simulink model "simulation_servo_agent"  (R2017b)
settings: Solver=FixedStepDiscrete  StartTime=0.0  StopTime=inf  FixedStep=Ts  MaxStep=1e-2  RelTol=1e-3  AbsTol=1e-3
PreLoadFcn:
  | pe_dc_motor_control_data;
values from neighbouring files (symbols this model uses):
  K = 0.00648887065107    [best_params.mat]    (also in parameter_twiddle_fast_kr.m = params(1))
  R = 5.66592438851    [best_params.mat]    (also in parameter_twiddle_fast_kr.m = params(2))
  Ts = 0.001    [best_params.mat]
undefined symbols (not defined in the file or in its folder): RawAcceleration, RawCurrent, RawPwm, RawRequestedVelocity, RawSupplyVoltage, RawTemperature, RawTimestamp, RawTorque, RawVelocity
libraries: fl_lib x21, nesl_utility x10, robotlib x8, dspstat3 x2, simulink x1, powerlib_meascontrol x1, commchan3 x1, sdl_lib x1
Description:
  | DC Motor Control
  | 
  | This example shows a cascade speed-control structure for a DC motor.
  | A PWM controlled four-quadrant Chopper is used to feed the DC motor.
  | The Control subsystem includes the outer speed-control loop, the inner
  | current-control loop, and the PWM generation. The total simulation
  | time (t) is 4 seconds. At t = 1.5 seconds, the load torque increases.
  | At t = 2.5 seconds, the reference speed is changed from 1000 rpm to
  | 2000 rpm.
  | 
  | Copyright 2016-2017 The MathWorks, Inc.
settings Model: Creator=The MathWorks, Inc.  LastModifiedBy=s158031
settings OptimizationCC: EnhancedBackFolding=on  PassReuseOutputArgsThreshold=0  MaxStackSize=64  OptimizeBlockOrder=speed  DifferentSizesBufferReuse=on
settings DebuggingCC: UnderspecifiedInitializationDetection=Classic  MergeDetectMultiDrivingBlocksExec=none  ParameterTunabilityLossMsg=error  SFUnexpectedBacktrackingDiag=warning  SFNoUnconditionalDefaultTransitionDiag=warning  SFExecutionAtInitializationDiag=none
settings HardwareCC: ProdBitPerPointer=32  ProdBitPerSizeT=32  ProdBitPerPtrDiffT=32  ProdLargestAtomicFloat=None  ProdIntDivRoundTo=Undefined  ProdEndianess=Unspecified  ProdWordSize=32  ProdHWDeviceType=Generic->Unspecified (assume 32-bit Generic)
settings SFSimCC: MATLABDynamicMemAlloc=off
settings RTWCC: SystemTargetFile=ert.tlc  HardwareBoard=Robot Operating System (ROS)  TemplateMakefile=ert_default_tmf  GenerateReport=on  Toolchain=Catkin  LaunchReport=on  TargetLang=C++
settings CodeAppCC: ForceParamTrailComments=on  OperatorAnnotations=on
settings ERTTargetCC: ERTCustomFileBanners=off  SupportContinuousTime=on  SupportNonInlinedSFcns=on  RemoveResetFunc=off  ModelStepFunctionPrototypeControlCompliant=off
settings ConfigComp: CovMetricSettings=dw  CovHtmlReporting=on  CovSaveCumulativeToWorkspaceVar=on  CovSaveSingleToWorkspaceVar=on  CovExternalEMLEnable=off
settings SimscapeCC: SimscapeLogName=simlog_pe_dc_motor_control  SimscapeLogLimitData=off

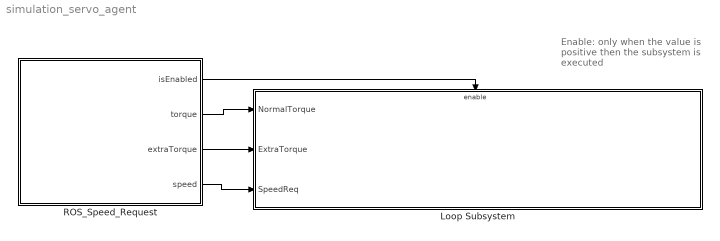
== system simulation_servo_agent ==
  note: Enable: only when the value is positive then the subsystem is executed
  Loop Subsystem : Subsystem
  ROS_Speed_Request : Subsystem
  wires:
  ROS_Speed_Request/2(torque) -> Loop Subsystem/1("NormalTorque ")
  ROS_Speed_Request/1(isEnabled) -> Loop Subsystem/Enable
  ROS_Speed_Request/3(extraTorque) -> Loop Subsystem/2(ExtraTorque)
  ROS_Speed_Request/4(speed) -> Loop Subsystem/3(SpeedReq)

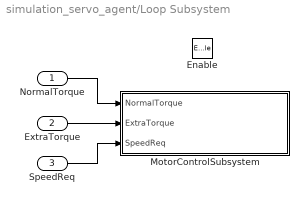
== system simulation_servo_agent/Loop Subsystem ==
  "NormalTorque " : Inport
  ExtraTorque : Inport  Port=2
  SpeedReq : Inport  Port=3
  Enable : EnablePort
  MotorControlSubsystem : Subsystem  TreatAsAtomicUnit=on
  wires:
  "NormalTorque "/1 -> MotorControlSubsystem/1(NormalTorque)
  SpeedReq/1 -> MotorControlSubsystem/3(SpeedReq)
  ExtraTorque/1 -> MotorControlSubsystem/2(ExtraTorque)

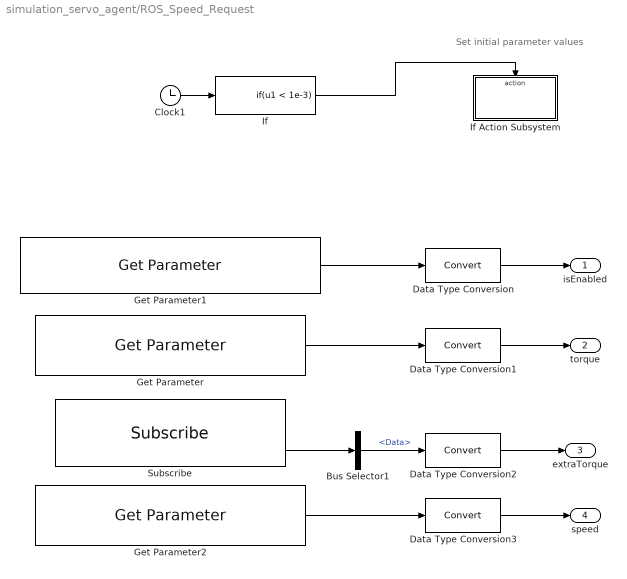
== system simulation_servo_agent/ROS_Speed_Request ==
  note: Set initial parameter values
  Bus Selector1 : BusSelector  OutputSignals=Data
  Clock1 : Clock
  Data Type Conversion{,1..3} (4 alike) : DataTypeConversion
  Get Parameter : robotlib/Get Parameter  SourceLibraryInfo=This block requires Robotics System Toolbox  ParameterSource=Select from ROS network  ParameterName=/simulation_servo_agent/add_torque/torque  ParameterType=double  ParameterMaxArrayLength=16  ParameterInitialValue=0.0  SampleTime=-1  ShowErrorCodeOutput=off  ModelName=simulation_servo_agent  BlockId=ParamGet_simulation_servo_agent_3318
      settings: SourceProductName=Robotics System Toolbox  SourceProductBaseCode=RO
  Get Parameter1 : robotlib/Get Parameter  SourceLibraryInfo=This block requires Robotics System Toolbox  ParameterSource=Select from ROS network  ParameterName=/simulation_servo_agent/update_velocity/isEnabled  ParameterType=boolean  ParameterMaxArrayLength=16  ParameterInitialValue=0.0  SampleTime=-1  ShowErrorCodeOutput=off  ModelName=simulation_servo_agent  BlockId=ParamGet_simulation_servo_agent_3398
      settings: SourceProductName=Robotics System Toolbox  SourceProductBaseCode=RO
  Get Parameter2 : robotlib/Get Parameter  SourceLibraryInfo=This block requires Robotics System Toolbox  ParameterSource=Select from ROS network  ParameterName=/simulation_servo_agent/update_velocity/speed  ParameterType=double  ParameterMaxArrayLength=16  ParameterInitialValue=0.0  SampleTime=-1  ShowErrorCodeOutput=off  ModelName=simulation_servo_agent  BlockId=ParamGet_simulation_servo_agent_3752
      settings: SourceProductName=Robotics System Toolbox  SourceProductBaseCode=RO
  If : If  IfExpression=u1 < 1e-3  ShowElse=off
  If Action Subsystem : Subsystem  TreatAsAtomicUnit=on
  Subscribe : robotlib/Subscribe  SourceLibraryInfo=This block requires Robotics System Toolbox  topicSource=Select from ROS network  topic=/conveyor_belt_agent/extra_torque  messageType=std_msgs/Float32  sampleTime=-1  messageQueueLength=1
      settings: SourceProductBaseCode=RO
  isEnabled : Outport
  torque : Outport  Port=2
  extraTorque : Outport  Port=3
  speed : Outport  Port=4
  wires:
  Get Parameter/1 -> Data Type Conversion1/1
  Get Parameter1/1 -> Data Type Conversion/1
  Data Type Conversion/1 -> isEnabled/1
  Clock1/1 -> If/1
  If/1 -> If Action Subsystem/Action
  Data Type Conversion1/1 -> torque/1
  Data Type Conversion3/1 -> speed/1
  Get Parameter2/1 -> Data Type Conversion3/1
  Subscribe/2 -> Bus Selector1/1
  Bus Selector1/1 -> Data Type Conversion2/1  "<Data>"
  Data Type Conversion2/1 -> extraTorque/1

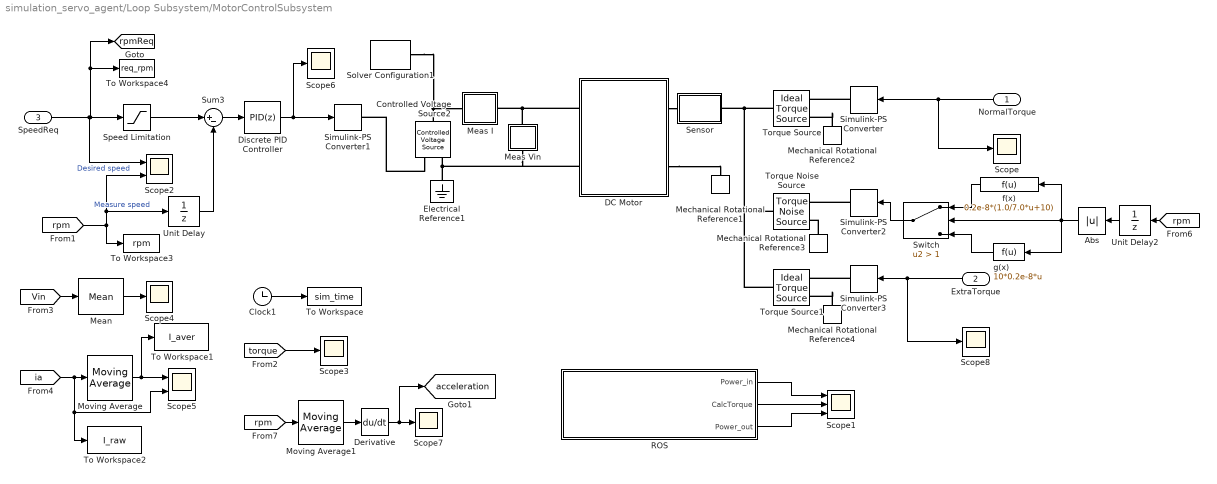
== system simulation_servo_agent/Loop Subsystem/MotorControlSubsystem ==
  NormalTorque : Inport
  ExtraTorque : Inport  Port=2
  SpeedReq : Inport  Port=3
  Abs : Abs
  Clock1 : Clock
  Controlled Voltage Source2 : fl_lib/Electrical/Electrical Sources/Controlled Voltage Source
  DC Motor : Subsystem
  Derivative : Derivative
  Discrete PID Controller : simulink/Continuous/PID Controller  Controller=PID  TimeDomain=Discrete-time  SampleTime=-1  IntegratorMethod=Forward Euler  FilterMethod=Forward Euler  Form=Parallel  UseFilter=on  ControllerParametersSource=internal  P=0.12  I=1.5  D=0.007  N=55  InitialConditionSource=internal  InitialConditionForIntegrator=0  InitialConditionForFilter=0  ExternalReset=none  LimitOutput=on  UpperSaturationLimit=11.1  LowerSaturationLimit=-11.1  LinearizeAsGain=off  AntiWindupMode=none  Kb=1  TrackingMode=off  Kt=1  PParamMin=[]  PParamMax=[]  IParamMin=[]  IParamMax=[]  DParamMin=[]  DParamMax=[]  NParamMin=[]  NParamMax=[]  KbParamMin=[]  KbParamMax=[]  KtParamMin=[]  KtParamMax=[]  POutMin=[]  POutMax=[]  IOutMin=[]  IOutMax=[]  DOutMin=[]  DOutMax=[]  NOutMin=[]  NOutMax=[]  KbOutMin=[]  KbOutMax=[]  KtOutMin=[]  KtOutMax=[]  IntegratorOutMin=[]  IntegratorOutMax=[]  FilterOutMin=[]  FilterOutMax=[]  SumOutMin=[]  SumOutMax=[]  SumI1OutMin=[]  SumI1OutMax=[]  SumI2OutMin=[]  SumI2OutMax=[]  SumI3OutMin=[]  SumI3OutMax=[]  SumDOutMin=[]  SumDOutMax=[]  SaturationOutMin=[]  SaturationOutMax=[]  IntegratorContinuousStateAttributes=''  IntegratorStateMustResolveToSignalObject=off  IntegratorRTWStateStorageClass=Auto  FilterContinuousStateAttributes=''  FilterStateMustResolveToSignalObject=off  FilterRTWStateStorageClass=Auto  DifferentiatorICPrevScaledInput=0  DifferentiatorOutMin=[]  DifferentiatorOutMax=[]  InitialConditionSetting=State (most efficient)  FilterDiffOutCoefMin=[]  FilterDiffOutCoefMax=[]  SumDenOutMin=[]  SumDenOutMax=[]  SumNumOutMin=[]  SumNumOutMax=[]  ReciprocalOutMin=[]  ReciprocalOutMax=[]  DivideOutMin=[]  DivideOutMax=[]  TunerSelectOption=Transfer Function Based (PID Tuner App)
  Electrical Reference1 : fl_lib/Electrical/Electrical Elements/Electrical Reference
      settings: SourceProductName=Foundation Library
  Mean : powerlib_meascontrol/Measurements/Mean  Freq=10  Vinit=0  Ts=Ts
  Meas I : Subsystem
  Meas Vin : Subsystem
  Mechanical Rotational Reference{1..4} (4 alike) : fl_lib/Mechanical/Rotational Elements/Mechanical Rotational Reference
      settings: SourceProductName=Foundation Library
  Moving Average : dspstat3/Moving Average  Method=Sliding window  SpecifyWindowLength=on  WindowLength=1000  ForgettingFactor=0.9  SimulateUsing=Code generation
  Moving Average1 : dspstat3/Moving Average  Method=Sliding window  SpecifyWindowLength=on  WindowLength=300  ForgettingFactor=0.9  SimulateUsing=Code generation
  ROS : Subsystem
  Scope{,3..4,6..8} (6 alike) : Scope
  Scope1 : Scope  NumInputPorts=3
  Scope2 : Scope  NumInputPorts=2
  Scope5 : Scope  NumInputPorts=2
  Sensor : Subsystem
  Simulink-PS Converter{,1..3} (4 alike) : nesl_utility/Simulink-PS Converter  PhysicalDomain=network_engine_domain  SubClassName=ps_input  LeftPortType=input  RightPortType=output  PseudoPeriodic=off  Frequencies=[]  NoiseDistribution=none  NoiseParameters=[]  Unit=1  AffineConversion=off  FilteringAndDerivatives=provide  SimscapeFilterOrder=1  InputFilterTimeConstant=0.001  UdotUserProvided=0
  Solver Configuration1 : nesl_utility/Solver Configuration  PhysicalDomain=network_engine_domain  SubClassName=solver  LeftPortType=input  RightPortType=generic  Accelerate=off  Tones=[]  Harmonics=[]  SimulateNoise=off  Profile=off  UseLocalSampling=off  EnableSwitchedLinearOptims=on  FrequencyDomain=off  UseCCode=off  RelTol=0.001  AbsTol=1e-06  MinStep=1e-09  ToWorkspace=off  RevertToSquareIcSolve=off  NumHomotopyIterations=100  PhasorMode=off  PhasorModeNumHarmonics=1  DoDC=off  ResidualTolerance=1e-09  UseLocalSolver=on  LocalSolverChoice=NE_BACKWARD_EULER_ADVANCER  LocalSolverSampleTime=Ts  DoFixedCost=on  MaxNonlinIter=3  MaxModeIter=2  LinearAlgebra=Sparse  DelaysMemoryBudget=1024  AutomaticFiltering=on  FilteringTimeConstant=0.001
  Speed Limitation : Saturate  UpperLimit=57  LowerLimit=-57
  Sum3 : Sum  Inputs=|+-
  Switch : Switch  Criteria=u2 > Threshold  Threshold=1
  To Workspace : ToWorkspace  VariableName=sim_time  SampleTime=-1
      settings: Save2DSignal=2-D array (concatenate along first dimension)
  To Workspace1 : ToWorkspace  VariableName=I_aver  SampleTime=-1
      settings: Save2DSignal=2-D array (concatenate along first dimension)
  To Workspace2 : ToWorkspace  VariableName=I_raw  SampleTime=-1
  To Workspace3 : ToWorkspace  VariableName=rpm  SampleTime=-1
      settings: Save2DSignal=2-D array (concatenate along first dimension)
  To Workspace4 : ToWorkspace  VariableName=req_rpm  SampleTime=-1
      settings: Save2DSignal=2-D array (concatenate along first dimension)
  Torque Source : fl_lib/Mechanical/Mechanical Sources/Ideal Torque Source
      settings: SourceProductName=Foundation Library
  Torque Source1 : fl_lib/Mechanical/Mechanical Sources/Ideal Torque Source
      settings: SourceProductName=Foundation Library
  Torque Noise Source : sdl_lib/Sources/Torque Noise Source  sample_time=1e-3 s  repeatability=3  user_seed=0  auto_seed=0
      settings: SourceProductName=Simscape Driveline  SourceProductBaseCode=LD
  Unit Delay : UnitDelay  SampleTime=Ts
  Unit Delay2 : UnitDelay  SampleTime=Ts
  f(x) : Fcn  Expr=0.2e-8*(1.0/7.0*u+10)
  g(x) : Fcn  Expr=10*0.2e-8*u
  tag scope: acceleration=global, rpmReq=global
  wires:
  NormalTorque/1 -> Simulink-PS Converter/1, Scope/1
  ROS/2(CalcTorque) -> Scope1/2
  ROS/1("Power_in ") -> Scope1/1
  ROS/3(Power_out) -> Scope1/3
  [Vin] -> Mean/1
  [ia] -> To Workspace2/1, Scope5/2, Moving Average/1
  Moving Average/1 -> To Workspace1/1, Scope5/1
  Mean/1 -> Scope4/1
  [rpm] -> To Workspace3/1, Unit Delay/1, Scope2/2  "Measure speed"
  Unit Delay/1 -> Sum3/2
  Clock1/1 -> To Workspace/1
  [torque] -> Scope3/1
  Speed Limitation/1 -> Sum3/1
  Sum3/1 -> Discrete PID Controller/1
  SpeedReq/1 -> [rpmReq], To Workspace4/1, Speed Limitation/1, Scope2/1  "Desired speed"
  Discrete PID Controller/1 -> Scope6/1, Simulink-PS Converter1/1
  [rpm] -> Moving Average1/1
  Derivative/1 -> [acceleration], Scope7/1
  Moving Average1/1 -> Derivative/1
  ExtraTorque/1 -> Scope8/1, Simulink-PS Converter3/1
  Switch/1 -> Simulink-PS Converter2/1
  f(x)/1 -> Switch/1
  [rpm] -> Unit Delay2/1
  Unit Delay2/1 -> Abs/1
  Abs/1 -> g(x)/1, f(x)/1, Switch/2
  g(x)/1 -> Switch/3
  connections:
  Meas Vin/LConn1 -- DC Motor/LConn1 -- Meas I/RConn1
  DC Motor/RConn1 -- Sensor/LConn1
  Simulink-PS Converter/RConn1 -- Torque Source/RConn1
  DC Motor/RConn2 -- Mechanical Rotational Reference1/LConn1
  Mechanical Rotational Reference2/LConn1 -- Torque Source/RConn2
  Electrical Reference1/LConn1 -- Controlled Voltage Source2/RConn2 -- DC Motor/LConn2 -- Meas Vin/RConn1
  Controlled Voltage Source2/LConn1 -- Solver Configuration1/RConn1 -- Meas I/LConn1
  Controlled Voltage Source2/RConn1 -- Simulink-PS Converter1/RConn1
  Torque Source/LConn1 -- Sensor/RConn1 -- Torque Source1/LConn1 -- Torque Noise Source/RConn1
  Simulink-PS Converter2/RConn1 -- Torque Noise Source/LConn1
  Mechanical Rotational Reference3/LConn1 -- Torque Noise Source/LConn2
  Simulink-PS Converter3/RConn1 -- Torque Source1/RConn1
  Mechanical Rotational Reference4/LConn1 -- Torque Source1/RConn2

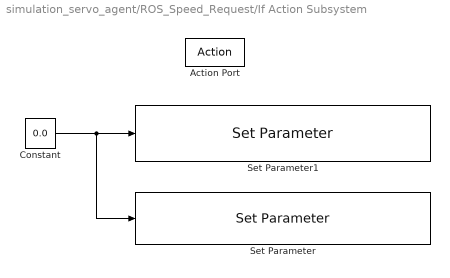
== system simulation_servo_agent/ROS_Speed_Request/If Action Subsystem ==
  Action Port : ActionPort  ActionType=then
  Constant : Constant  Value=0.0
  Set Parameter : robotlib/Set Parameter  SourceLibraryInfo=This block requires Robotics System Toolbox  ParameterSource=Select from ROS network  ParameterName=/simulation_servo_agent/update_velocity/isEnabled  ParameterType=double  ModelName=simulation_servo_agent  BlockId=ParamSet_simulation_servo_agent_3446
      settings: SourceProductName=Robotics System Toolbox  SourceProductBaseCode=RO
  Set Parameter1 : robotlib/Set Parameter  SourceLibraryInfo=This block requires Robotics System Toolbox  ParameterSource=Select from ROS network  ParameterName=/simulation_servo_agent/update_velocity/speed  ParameterType=double  ModelName=simulation_servo_agent  BlockId=ParamSet_simulation_servo_agent_3447
      settings: SourceProductName=Robotics System Toolbox  SourceProductBaseCode=RO
  wires:
  Constant/1 -> Set Parameter/1, Set Parameter1/1

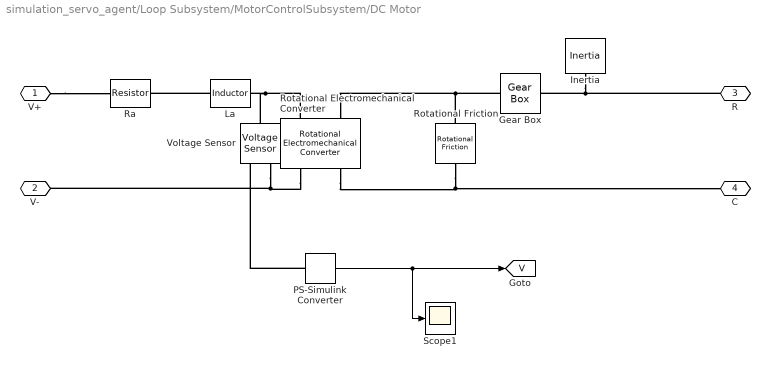
== system simulation_servo_agent/Loop Subsystem/MotorControlSubsystem/DC Motor ==
  Gear Box : fl_lib/Mechanical/Mechanisms/Gear Box  ratio=258.5  t_in_specify=off  t_in_priority=None  t_in=0 N*m  t_in_nominal_specify=off  t_in_nominal_unit=N*m  t_in_nominal_value=1  t_out_specify=off  t_out_priority=None  t_out=0 N*m  t_out_nominal_specify=off  t_out_nominal_unit=N*m  t_out_nominal_value=1
  Inertia : fl_lib/Mechanical/Rotational Elements/Inertia  inertia=J kg*m^2  w_specify=off  w_priority=High  w=0 rad/s  w_nominal_specify=off  w_nominal_unit=rad/s  w_nominal_value=1  t_specify=off  t_priority=None  t=0 N*m  t_nominal_specify=off  t_nominal_unit=N*m  t_nominal_value=1
      settings: SourceProductName=Foundation Library
  La : fl_lib/Electrical/Electrical Elements/Inductor  l=L H  r=0 Ohm  g=1e-9 1/Ohm  i_specify=off  i_priority=None  i=0 A  i_nominal_specify=off  i_nominal_unit=A  i_nominal_value=1  v_specify=off  v_priority=None  v=0 V  v_nominal_specify=off  v_nominal_unit=V  v_nominal_value=1  i_L_specify=on  i_L_priority=High  i_L=0 A  i_L_nominal_specify=off  i_L_nominal_unit=A  i_L_nominal_value=1
      settings: SourceProductName=Foundation Library
  PS-Simulink Converter : nesl_utility/PS-Simulink Converter  PhysicalDomain=network_engine_domain  SubClassName=ps_output  LeftPortType=input  RightPortType=output  PseudoPeriodic=off  Frequencies=[]  Unit=1  AffineConversion=off
  Ra : fl_lib/Electrical/Electrical Elements/Resistor  R=R Ohm  i_specify=off  i_priority=None  i=0 A  i_nominal_specify=off  i_nominal_unit=A  i_nominal_value=1  v_specify=off  v_priority=None  v=0 V  v_nominal_specify=off  v_nominal_unit=V  v_nominal_value=1
      settings: SourceProductName=Foundation Library
  Rotational Electromechanical Converter : fl_lib/Electrical/Electrical Elements/Rotational Electromechanical Converter  K=K V/(rad/s)  i_specify=off  i_priority=None  i=0 A  i_nominal_specify=off  i_nominal_unit=A  i_nominal_value=1  v_specify=off  v_priority=None  v=0 V  v_nominal_specify=off  v_nominal_unit=V  v_nominal_value=1  t_specify=off  t_priority=None  t=0 N*m  t_nominal_specify=off  t_nominal_unit=N*m  t_nominal_value=1  w_specify=off  w_priority=None  w=0 rad/s  w_nominal_specify=off  w_nominal_unit=rad/s  w_nominal_value=1
      settings: SourceProductName=Foundation Library
  Rotational Friction : fl_lib/Mechanical/Rotational Elements/Rotational Friction  brkwy_trq=C N*m  brkwy_vel=1e-5 rad/s  Col_trq=C N*m  visc_coef=F N*m/(rad/s)  w_specify=off  w_priority=None  w=0 rad/s  w_nominal_specify=off  w_nominal_unit=rad/s  w_nominal_value=1  t_specify=off  t_priority=None  t=0 N*m  t_nominal_specify=off  t_nominal_unit=N*m  t_nominal_value=1
      settings: SourceProductName=Simscape
  Scope1 : Scope
  Voltage Sensor : fl_lib/Electrical/Electrical Sensors/Voltage Sensor
  V+ : PMIOPort  Port=1  Side=Left
  V- : PMIOPort  Port=2  Side=Left
  R : PMIOPort  Port=3  Side=Right
  C : PMIOPort  Port=4  Side=Right
  tag scope: V=global
  wires:
  PS-Simulink Converter/1 -> Scope1/1, [V]
  connections:
  Rotational Electromechanical Converter/RConn1 -- Voltage Sensor/RConn2 -- V-/RConn1
  V+/RConn1 -- Ra/LConn1
  Rotational Electromechanical Converter/RConn2 -- Rotational Friction/RConn1 -- C/RConn1
  Gear Box/LConn1 -- Rotational Electromechanical Converter/LConn2 -- Rotational Friction/LConn1
  R/RConn1 -- Inertia/LConn1 -- Gear Box/RConn1
  Rotational Electromechanical Converter/LConn1 -- Voltage Sensor/LConn1 -- La/RConn1
  La/LConn1 -- Ra/RConn1
  PS-Simulink Converter/LConn1 -- Voltage Sensor/RConn1

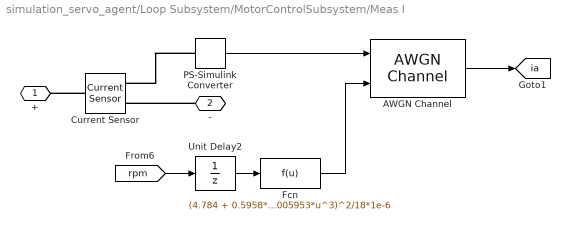
== system simulation_servo_agent/Loop Subsystem/MotorControlSubsystem/Meas I ==
  AWGN Channel : commchan3/AWGN Channel  InputProcessing=Columns as channels (frame based)  seed=67  noiseMode=Variance from port  EbNodB=10  EsNodB=10  SNRdB=10  bitsPerSym=1  Ps=1  Tsym=1  variance=1
  Current Sensor : fl_lib/Electrical/Electrical Sensors/Current Sensor
      settings: SourceProductName=Foundation Library
  Fcn : Fcn  Expr=(4.784 + 0.5958*u -0.02393*u^2+0.0005953*u^3)^2/18*1e-6
  PS-Simulink Converter : nesl_utility/PS-Simulink Converter  PhysicalDomain=network_engine_domain  SubClassName=ps_output  LeftPortType=input  RightPortType=output  PseudoPeriodic=off  Frequencies=[]  Unit=1  AffineConversion=off
  Unit Delay2 : UnitDelay  SampleTime=Ts
  + : PMIOPort  Port=1  Side=Left
  - : PMIOPort  Port=2  Side=Right
  tag scope: ia=global
  wires:
  AWGN Channel/1 -> [ia]
  [rpm] -> Unit Delay2/1
  Fcn/1 -> AWGN Channel/2
  Unit Delay2/1 -> Fcn/1
  PS-Simulink Converter/1 -> AWGN Channel/1
  connections:
  PS-Simulink Converter/LConn1 -- Current Sensor/RConn1
  Current Sensor/LConn1 -- +/RConn1
  -/RConn1 -- Current Sensor/RConn2

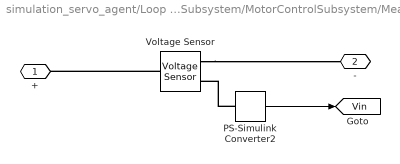
== system simulation_servo_agent/Loop Subsystem/MotorControlSubsystem/Meas Vin ==
  PS-Simulink Converter2 : nesl_utility/PS-Simulink Converter  PhysicalDomain=network_engine_domain  SubClassName=ps_output  LeftPortType=input  RightPortType=output  PseudoPeriodic=off  Frequencies=[]  Unit=V  AffineConversion=off
  Voltage Sensor : fl_lib/Electrical/Electrical Sensors/Voltage Sensor
      settings: SourceProductName=Foundation Library
  + : PMIOPort  Port=1  Side=Left
  - : PMIOPort  Port=2  Side=Right
  tag scope: Vin=global
  wires:
  PS-Simulink Converter2/1 -> [Vin]
  connections:
  Voltage Sensor/LConn1 -- +/RConn1
  PS-Simulink Converter2/LConn1 -- Voltage Sensor/RConn1
  Voltage Sensor/RConn2 -- -/RConn1

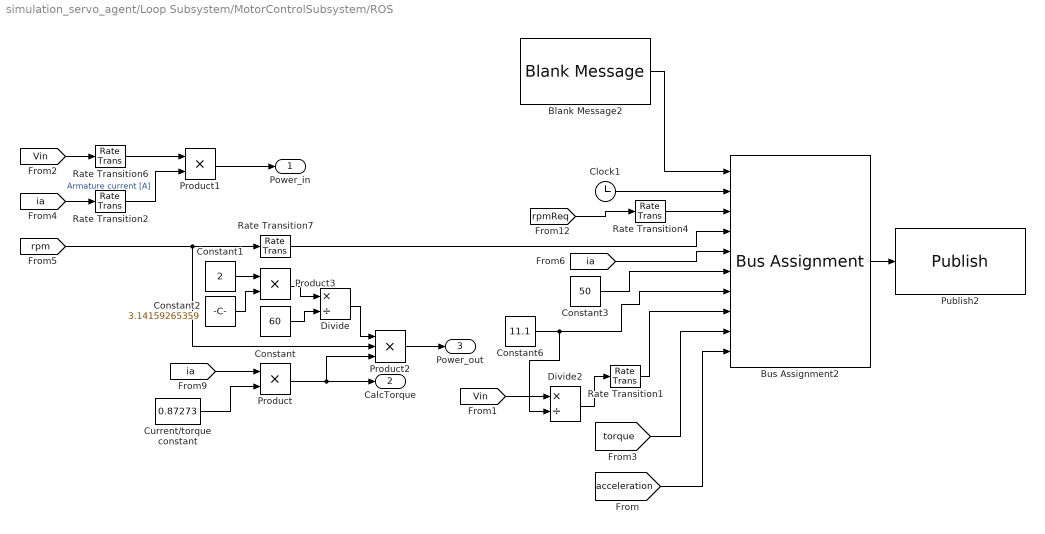
== system simulation_servo_agent/Loop Subsystem/MotorControlSubsystem/ROS ==
  Blank Message2 : robotlib/Blank Message  SourceLibraryInfo=This block requires Robotics System Toolbox  messageType=dobot/motor_raw_data  SampleTime=inf
      settings: SourceProductBaseCode=RO
  Bus Assignment2 : BusAssignment  AssignedSignals=RawTimestamp,RawRequestedVelocity,RawVelocity,RawCurrent,RawTemperature,RawSupplyVoltage,RawPwm,RawTorque,RawAcceleration
  Clock1 : Clock
  Constant : Constant  Value=60
  Constant1 : Constant  Value=2
  Constant2 : Constant  Value=3.14159265359
  Constant3 : Constant  Value=50
  Constant6 : Constant  Value=11.1
  Current/torque constant : Constant  Value=0.87273
  Divide : Product  Inputs=*/
  Divide2 : Product  Inputs=*/
  Product : Product
  Product1 : Product
  Product2 : Product  Inputs=3
  Product3 : Product
  Publish2 : robotlib/Publish  SourceLibraryInfo=This block requires Robotics System Toolbox  topicSource=Specify your own  topic=/simulation_servo_agent/motor_raw_data  messageType=dobot/motor_raw_data  messageQueueLength=105
      settings: SourceProductBaseCode=RO
  Rate Transition{1..2,4,6..7} (5 alike) : RateTransition
  "Power_in " : Outport  InitialOutput=[10]
  CalcTorque : Outport  Port=2
  Power_out : Outport  Port=3
  wires:
  Divide/1 -> Product2/1
  Rate Transition2/1 -> Product1/2  "Armature current [A]"
  [ia] -> Product/1
  Blank Message2/1 -> Bus Assignment2/1
  Clock1/1 -> Bus Assignment2/2
  Product/1 -> Product2/3, CalcTorque/1
  Constant1/1 -> Product3/1
  [rpmReq] -> Rate Transition4/1
  Constant/1 -> Divide/2
  Rate Transition4/1 -> Bus Assignment2/3
  Constant3/1 -> Bus Assignment2/6
  [Vin] -> Rate Transition6/1
  Bus Assignment2/1 -> Publish2/1
  Rate Transition7/1 -> Bus Assignment2/4
  Current/torque constant/1 -> Product/2
  Constant2/1 -> Product3/2
  [rpm] -> Product2/2, Rate Transition7/1
  Product3/1 -> Divide/1
  Product2/1 -> Power_out/1
  Rate Transition6/1 -> Product1/1
  Product1/1 -> "Power_in "/1
  [ia] -> Rate Transition2/1
  [ia] -> Bus Assignment2/5
  Constant6/1 -> Bus Assignment2/7, Divide2/2
  Rate Transition1/1 -> Bus Assignment2/8
  Divide2/1 -> Rate Transition1/1
  [Vin] -> Divide2/1
  [acceleration] -> Bus Assignment2/10
  [torque] -> Bus Assignment2/9

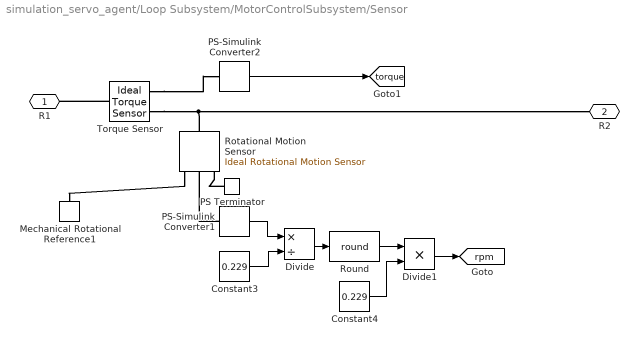
== system simulation_servo_agent/Loop Subsystem/MotorControlSubsystem/Sensor ==
  Constant3 : Constant  Value=0.229
  Constant4 : Constant  Value=0.229
  Divide : Product  Inputs=*/
  Divide1 : Product  Inputs=**
  Mechanical Rotational Reference1 : fl_lib/Mechanical/Rotational Elements/Mechanical Rotational Reference
      settings: SourceProductName=Foundation Library
  PS Terminator : fl_lib/Physical Signals/Sinks/PS Terminator
      settings: SourceProductName=Foundation Library
  PS-Simulink Converter1 : nesl_utility/PS-Simulink Converter  PhysicalDomain=network_engine_domain  SubClassName=ps_output  LeftPortType=input  RightPortType=output  PseudoPeriodic=off  Frequencies=[]  Unit=rpm  AffineConversion=off
  PS-Simulink Converter2 : nesl_utility/PS-Simulink Converter  PhysicalDomain=network_engine_domain  SubClassName=ps_output  LeftPortType=input  RightPortType=output  PseudoPeriodic=off  Frequencies=[]  Unit=N*m  AffineConversion=off
  Rotational Motion Sensor : fl_lib/Mechanical/Mechanical Sensors/Ideal Rotational Motion Sensor  offset=0 rad
      settings: SourceProductName=Foundation Library
  Round : Rounding  Operator=round
  Torque Sensor : fl_lib/Mechanical/Mechanical Sensors/Ideal Torque Sensor
      settings: SourceProductName=Foundation Library
  R1 : PMIOPort  Port=1  Side=Left
  R2 : PMIOPort  Port=2  Side=Right
  tag scope: rpm=global, torque=global
  wires:
  PS-Simulink Converter2/1 -> [torque]
  PS-Simulink Converter1/1 -> Divide/1
  Divide/1 -> Round/1
  Round/1 -> Divide1/1
  Constant3/1 -> Divide/2
  Constant4/1 -> Divide1/2
  Divide1/1 -> [rpm]
  connections:
  Rotational Motion Sensor/RConn1 -- Mechanical Rotational Reference1/LConn1
  Torque Sensor/LConn1 -- R1/RConn1
  Torque Sensor/RConn2 -- PS-Simulink Converter2/LConn1
  PS-Simulink Converter1/LConn1 -- Rotational Motion Sensor/RConn2
  PS Terminator/LConn1 -- Rotational Motion Sensor/RConn3
  Torque Sensor/RConn1 -- R2/RConn1 -- Rotational Motion Sensor/LConn1
